simulink model "PI Controller Vector Controlled IM Drive"  (R2020b)
settings: Solver=ode4  StartTime=0.0  StopTime=5  RelTol=1e-3
InitFcn:
  | %clear;
  | %clc;
  | 
  | %Motor Parameters
  | r1 = 1.405;
  | l1  = 0.005839;
  | r2 = 1.395;
  | l2 = 0.005839;
  | Lm = 0.1722;
  | J = 0.0131;
  | 
  | %Motor Rated Values
  | Vrat = 400;
  | frat = 50;
  | 
  | x1 = 2*pi*frat*l1;
  | x2 = 2*pi*frat*l2;
  | Xm = 2*pi*frat*Lm;
  | Prat = 4*1000;
  | Nrat = 1430;
  | P = 4;
  | Ns = 120*frat/P;
  | nrat = Nrat*2*pi/60;
  | ns = Ns*2*pi/60;
  | srat = (Ns-Nrat)/Ns;
  | 
  | E1 = Vrat/sqrt(3); %phase voltage
  | IL = E1/( (r1 + (1i*x1) ) + ( ( (1i*x2) +(r2/srat) )*1i*Xm / ( (1i*Xm) + (1i*x2) + (r2/srat) ) ) );
  | E2 = E1 - (IL*(r1 + (1i*x1) ) );
  | Trat = (3/(ns))*srat*abs(E2)*abs(E2)*r2/((r2*r2) + (srat*srat*x2*x2));
  | %Trat = Prat/nrat;
  | 
  | %System Variables
  | Tsys = (1e-6);
  | Ts = (100e-6);
  | freq = 50;
  | ws = freq*2*pi;
  | 
  | m=1*freq/50;
  | %m = 1 * (freq/50);
  | Vbus = (400*sqrt(2)*2/sqrt(3)) / (1.15);
  | 
  | Vref = (Vbus*sqrt(3)/2) * m;
  | delay = Ts/Tsys;
  | 
  | % Motor Starting Parameters
  | inc_time = 0.1;
  | 
  | %Motor Loading time
  | load_time = 0;
  | 
  | %No. of Hybrid Zones
  | numzones = 3;
  | 
  | %Load ML model Weights
  | 
  | W1R_s1 = readmatrix('Regression Weights\W1_subnet1_tmp_odd_90.xlsx');
  | b1R_s1 = readmatrix('Regression Weights\b1_subnet1_tmp_odd_90.xlsx');
  | W1R_s2 = readmatrix('Regression Weights\W1_subnet2_tmp_odd_90.xlsx');
  | b1R_s2 = readmatrix('Regression Weights\b1_subnet2_tmp_odd_90.xlsx');
  | ... (+35 lines)
undefined symbols (not defined in the file): DiscIntNeverNeededParam
libraries: powerlib x21, simulink x19, pid_lib x4, powerlib_meascontrol x4, simulink_extras x2
(part 3 of 3)

== matlab function PI Controller Vector Controlled IM Drive/Space Vector PWM based VSI 1/Switching Times and Sector/Switch Times and Sequence Calculation ==
  data: Vref input; angle input; Ts input; Vbus input; sector output
function sector  = fcn(Vref, angle, Ts, Vbus)
    
    numzones = 3;
    %     Using ML Models 
    m = (2/sqrt(3))*(Vref/Vbus);
    theta = rem(angle, (pi/3));
    flag = 0;
    if numzones == 1
        flag = 1;
    end
    
    %Switching times calculation of different vectors
    if m <= 1                % Linear modulation (Overmodulation mode 0)
        n2 = Vref*cos( theta );
        n1 = Vref*cos( (pi/3) - theta );

        T1 = (2*Ts/(3*Vbus)) * ((-n1) + (2*n2));
        T2 = (2*Ts/(3*Vbus)) * ((2*n1) - n2);
        T0 = Ts-(T1+T2);
        flag = 1;
        
    elseif m<=1.05      % Overmodulation mode I
        alpha_t = (pi/6) - acos(1/m);
        alpha_t = alpha_t/2;
        if theta > alpha_t && theta < (pi/3) - alpha_t
            T1 = (sin( (pi/3) - theta ) / ( sin( (pi/3) - theta ) + sin( theta ) ) ) * Ts;
            T2 = Ts-T1;
            T0=0;
        else
            n2 = Vref*cos( theta );
            n1 = Vref*cos( (pi/3) - theta );
            T1 = (2*Ts/(3*Vbus)) * ((-n1) + (2*n2));
            T2 = (2*Ts/(3*Vbus)) * ((2*n1) - n2);
            T0 = Ts-(T1+T2);
            flag = 1;
        end
        
    elseif m <= 1.10    % Overmodulation mode II
        alpha_h = (pi/6) - acos(1/m);
        if theta <= alpha_h
            T1 = Ts;
            T2=0;
            T0=0;
            
        elseif theta > alpha_h && theta < (pi/3) - alpha_h
            T1 = (sin( (pi/3) - theta ) / ( sin( (pi/3) - theta ) + sin( theta ) ) ) * Ts;
            T2 = Ts-T1;
            T0=0;
            
        else
            T1 = 0;
            T2 = Ts;
            T0 = 0;
        end
        
    else        % Six Step Mode
        if theta <= (pi/6)
            T1 = Ts;
            T2 = 0;
            T0 = 0;
        else
            T1 = 0;
            T2 = Ts;
            T0 = 0;
        end
        
    end
    
    if flag == 1
        % Switching Sequence Determination
        Q1 = (cos(theta) - (Vref/Vbus)) * T1;
        Q2 = (cos( (pi/3) - theta) - (Vref/Vbus)) * T2;
        Q0 = - (Vref/Vbus)*T0;
        D = sin(theta) * T1;

        %Error Functions (Squared) for Different Switching Sequences
        F_0127 = ( (1/3) * ( (0.5*Q0).^2 ) * T0 / (2*Ts) ) + ( (1/3) * ( ( (0.5*Q0).^2 ) + ( 0.5*Q0* ( (0.5*Q0) + Q1 ) ) + ( ( 1* ( (0.5*Q0) + Q1 ) ).^2) ) * (T1/Ts) ) + ( (1/3) * ( ( ( (0.5*Q0) + Q1).^2) - ( ( (0.5*Q0) + Q1) * (0.5*Q0) ) + ( (0.5*Q0).^2 ) ) * (T2/Ts) ) + ( (1/3) * ( (0.5*Q0).^2 ) * ( T0 / (2*Ts) ) ) + ( (1/3) * (D.^2) * ( (T1+T2) / Ts ) );

        F_012 = ( (4/27) * (Q0.^2) * (T0/Ts) ) + ( (4/27) * ( (Q0.^2) + ( Q0*(Q0+Q1) ) + ( (Q0+Q1).^2 ) ) * (T1/Ts) ) + ( (4/27) * ( (Q0+Q1).^2 ) * (T2/Ts) ) + ( (4/27) * (D.^2) * ( (T1+T2) / Ts) );

        F_721 = ( (4/27) * (Q0.^2) * (T0/Ts) ) + ( (4/27) * ( (Q0.^2) + ( Q0*(Q0+Q2) ) + ( (Q0+Q2).^2 ) ) * (T2/Ts) ) + ( (4/27) * ( (Q0+Q2).^2 ) * (T1/Ts) ) + ( (4/27) * (D.^2) * ( (T1+T2) / Ts) );

        F_0121 = ( (1/3) * (Q0.^2) * (T0/Ts) ) + ( (1/3) * ( (Q0.^2) + ( Q0*( Q0 + (0.5*Q1) ) ) + ( ( Q0 + (0.5*Q1) ).^2 ) ) * ( T1 / (2*Ts) ) ) + ( (1/3) * ( ( ( Q0 + (0.5*Q1) ).^2 ) - ( ( Q0 + (0.5*Q1) ) * (0.5*Q1) ) + ( (0.5*Q1).^2 ) ) * (T2/Ts) ) + ( (1/3) * ( (0.5*Q1).^2 ) * (T1 / (2*Ts) ) ) + ( (1/3) * ( (0.5*D).^2 ) * ( (T1+T2) / Ts ) );

        F_7212 = ( (1/3) * (Q0.^2) * (T0/Ts) ) + ( (1/3) * ( (Q0.^2) + ( Q0*( Q0 + (0.5*Q2) ) ) + ( ( Q0 + (0.5*Q2) ).^2 ) ) * ( T2 / (2*Ts) ) ) + ( (1/3) * ( ( ( Q0 + (0.5*Q2) ).^2 ) - ( ( Q0 + (0.5*Q2) ) * (0.5*Q2) ) + ( (0.5*Q2).^2 ) ) * (T1/Ts) ) + ( (1/3) * ( (0.5*Q2).^2 ) * (T2 / (2*Ts) ) ) + ( (1/3) * ( (0.5*D).^2 ) * ( (T1+T2) / Ts ) );

        F_1012 = ( (1/3) * ( ( 0.5*Q1).^2 ) * (T1 / (2*Ts) ) ) + ( (1/3) * ( ( (0.5*Q1).^2 ) + ( 0.5*Q1*( (0.5*Q1) + Q0 ) ) + ( ( (0.5*Q1) + Q0 ).^2 ) ) * (T0/Ts) ) + ( (1/3) * ( ( ( (0.5*Q1) + Q0 ).^2 ) - ( ( (0.5*Q1) + Q0 )*Q2 ) + (Q2.^2) ) * ( T1 / (2*Ts) ) ) + ( (1/3) * (Q2.^2) * (T2/Ts) ) + ( (1/3) * ( (0.5*D).^2 ) * ( T1 / (2*Ts) ) ) + ( ( (0.5*D).^2 ) * (T0/Ts) ) + ( (1/3) * ( ( (0.5*D).^2 ) + ( (0.5*D) * D ) + (D.^2) ) * ( T1 / (2*Ts) ) ) + ( (1/3) * (D.^2) * (T2/Ts) );

        F_2721 = ( (1/3) * ( ( 0.5*Q2).^2 ) * (T2 / (2*Ts) ) ) + ( (1/3) * ( ( (0.5*Q2).^2 ) + ( 0.5*Q2*( (0.5*Q2) + Q0 ) ) + ( ( (0.5*Q2) + Q0 ).^2 ) ) * (T0/Ts) ) + ( (1/3) * ( ( ( (0.5*Q2) + Q0 ).^2 ) - ( ( (0.5*Q2) + Q0 )*Q1 ) + (Q1.^2) ) * ( T2 / (2*Ts) ) ) + ( (1/3) * (Q1.^2) * (T1/Ts) ) + ( (1/3) * ( (0.5*D).^2 ) * ( T2 / (2*Ts) ) ) + ( ( (0.5*D).^2 ) * (T0/Ts) ) + ( (1/3) * ( ( (0.5*D).^2 ) + ( (0.5*D) * D ) + (D.^2) ) * ( T2 / (2*Ts) ) ) + ( (1/3) * (D.^2) * (T1/Ts) );
        
        if numzones == 1
            F = [F_0127];
            
        elseif numzones == 3
            %For Three Zone Hybrid PWM
            F = [F_0127, F_0121, F_7212];
            
        elseif numzones == 5
            %For Five Zone Hybrid PWM
            F = [F_0127, F_0121, F_7212, F_1012, F_2721];
        
        elseif numzones == 7
            %For Seven Zone Hybrid PWM
            F = [F_0127, F_0121, F_7212, F_1012, F_2721, F_012, F_721];
            
        else
            F = F_0127;
        end
        
        [~, idx] = min(F);

        if idx == 1
            switchseq = "0127";
        elseif idx == 2
            switchseq = "0121";
        elseif idx == 3
            switchseq = "7212";
        elseif idx == 4
            switchseq = "1012";
        elseif idx == 5
            switchseq = "2721";
        elseif idx == 6
            switchseq = "012";
        elseif idx == 7
            switchseq = "721";
        else
            switchseq = "0127";
        end
        
    else
        if theta < (pi/6)
            switchseq = "0121";
        else
            switchseq = "7212";
        end
    end
    
    % Switching Times calculation of switches
    Vsamp = Vref*exp(1i*angle);
    
    V1 = Vbus*exp(1i*0);
    V2 = Vbus*exp(1i*(pi/3));
    V3 = Vbus*exp(1i*(2*pi/3));
    V4 = Vbus*exp(1i*(3*pi/3));
    V5 = Vbus*exp(1i*(4*pi/3));
    V6 = Vbus*exp(1i*(5*pi/3));

    V = [V1; V2; V3; V4; V5; V6];
    V = V - Vsamp;
    [~, minVidx] = mink(V, 2);

%         minVidx = minVidx(:, 1);

    if max(minVidx) == 6 && min(minVidx) == 1
        minVidx = 6;
    else
        minVidx = min(minVidx);
    end
    
    sector = minVidx;
    
    if switchseq == "0127"
        swseq = 1;
    elseif switchseq == "0121"
        swseq = 2;
    elseif switchseq == "7212"
        swseq = 3;
    elseif switchseq == "1012"
        swseq = 4;
    elseif switchseq == "2721"
        swseq = 5;
    elseif switchseq == "012"
        swseq = 6;
    elseif switchseq == "721"
        swseq = 7;
    else
        swseq = 1;
    end
%     
%     %Using NN to predict switch times
%     
%     %Loading Necessary weight matrices
%     W1 = evalin('base', 'W1R');
%     b1 = evalin('base', 'b1R');
%     W2 = evalin('base', 'W2R');
%     b2 = evalin('base', 'W2R');
%     
%     %Predicting Switch Times
%     X = [m angle];
% %     y1 = zeros(1, size(b1, 1));
% %     y2 = zeros(1, size(b2, 2));
%     
%     y = X*(W1');
%     y = y + b1';      %Passing through 1st Layer (Hidden)
%     y = tanh(y);                  %Applying Activation Function (tanh)
%     
%     y = y*W2';
%     y = y+b2';        %Passing through 2nd Layer (Output)
%     y = 1./(1+exp(-y));      %Applying Activation Function (sigmoid)
%     
%     %Allocating Switch Times
%     S1 = y(1)*Ts;
%     S3 = y(2)*Ts;
%     S5 = y(3)*Ts;
    
end

== matlab function PI Controller Vector Controlled IM Drive/Space Vector PWM based VSI 1/Switching Times and Sector/m ==
  data: Vref input; m output; Vbus input
function m = fcn(Vref, Vbus)
    m = (2/sqrt(3)) * Vref/Vbus;
end

== matlab function PI Controller Vector Controlled IM Drive/3 Phase Induction Machine/MATLAB Function1 ==
  data: is_alpha input; is_beta input; i_sd output; theta_rf input; i_sq output
function [i_sd, i_sq] = fcn(is_alpha, is_beta, theta_rf)
    i_sd = (is_alpha*cos(theta_rf)) + (is_beta*sin(theta_rf));
    i_sq = (is_beta*cos(theta_rf)) - (is_alpha*sin(theta_rf));
end

== matlab function PI Controller Vector Controlled IM Drive/MATLAB Function ==
  data: abc input; dq0 output; wt input
function dq0 = fcn(abc, wt)
    matrix = [
            cos(wt) cos(wt-(2*pi/3)) cos(wt+(2*pi/3));
            -sin(wt) -sin(wt-(2*pi/3)) -sin(wt+(2*pi/3))
            0.5 0.5 0.5
            ];
    dq0 = matrix*abc;
end

== matlab function PI Controller Vector Controlled IM Drive/Space Vector PWM based VSI 1/3 Phase VSI/MATLAB Function ==
  data: iter input; iter output; arr input size=[1 3]; Va input; Vb input; Vc input; Ts input; Tsys input; arr output
function [iter, arr] = fcn(iter, arr, Va, Vb, Vc, Ts, Tsys)
    if iter == Ts/Tsys
        iter=0;
        arr = zeros(1,3);
    end
    arr(1, 1) = arr(1, 1) + (Va*Tsys/Ts);
    arr(1, 2) = arr(1, 2) + (Vb*Tsys/Ts);
    arr(1, 3) = arr(1, 3) + (Vc*Tsys/Ts);
    iter = iter+1;
end

== matlab function PI Controller Vector Controlled IM Drive/Space Vector PWM based VSI 1/Gating Pulse Generator/Gate Pulse Generator for 0121 Sequence/For Even Sector/MATLAB Function ==
  data: S1 input; S1 output; S3 input; S5 input; S3 output; S5 output; addtime output; addidx output
function [S1, S3, S5, addtime,addidx] = fcn(S1, S3, S5)
    S = [S1 S3 S5];
    [~, idx] = mink([S1 S3 S5], 3);
    
    addtime = (S(idx(2)) - S(idx(1)))/2;
    addidx = idx(2);
    S(idx(2)) = S(idx(2)) - addtime;
    
    S1 = S(1);
    S3 = S(2);
    S5 = S(3);
end

== matlab function PI Controller Vector Controlled IM Drive/Space Vector PWM based VSI 1/Gating Pulse Generator/Gate Pulse Generator for 0121 Sequence/For Odd Sector/MATLAB Function ==
  data: S1 input; S1 output; S3 input; S5 input; S3 output; S5 output; subtime output; subidx output
function [S1, S3, S5, subtime,subidx] = fcn(S1, S3, S5)
    S = [S1 S3 S5];
    [~, idx] = mink([S1 S3 S5], 3);
    
    S(idx(2)) = (S(idx(2)) + S(idx(3)))/2;
    
    subidx = idx(2);
    subtime = S(idx(3)) - S(idx(2));
    
    S1 = S(1);
    S3 = S(2);
    S5 = S(3);
end

== matlab function PI Controller Vector Controlled IM Drive/Space Vector PWM based VSI 1/Gating Pulse Generator/Gate Pulse Generator for 0127 Sequence 1/For Even Sector/MATLAB Function ==
  data: S1 input; S1 output; S3 input; S5 input; S3 output; S5 output; addtime output; addidx output
function [S1, S3, S5, addtime,addidx] = fcn(S1, S3, S5)
    S = [S1 S3 S5];
    [~, idx] = mink([S1 S3 S5], 3);
    
    addtime = (S(idx(3)) - S(idx(2)))/2;
    addidx = idx(3);
    S(idx(3)) = S(idx(3)) - addtime;
    
    S1 = S(1);
    S3 = S(2);
    S5 = S(3);
end
